simulink model "fm_modulation"  (R2023a)
settings: Solver=VariableStepAuto  StartTime=0.0  StopTime=.1  RelTol=1e-3
settings Model: Creator=USER  LastModifiedBy=USER

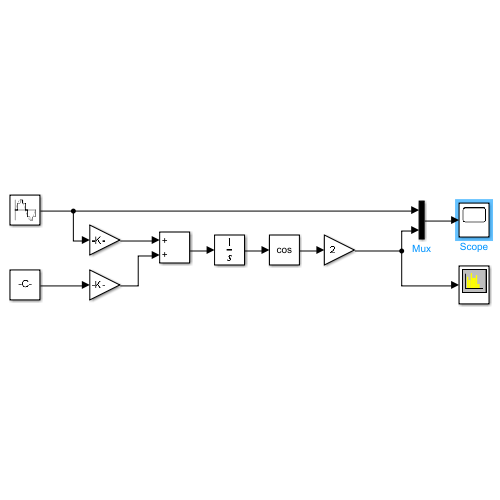
[thumbnail: Simulink's stored preview of the top-level diagram]
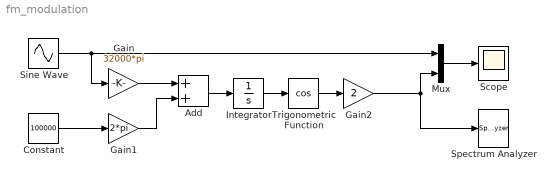
== system fm_modulation ==
  Add : Sum
  Constant : Constant  Value=100000
  Gain : Gain  Gain=32000*pi
  Gain1 : Gain  Gain=2*pi
  Gain2 : Gain  Gain=2
  Integrator : Integrator
  Mux : Mux  Inputs=2
  Scope : Scope
  Sine Wave : Sin  Amplitude=2  Frequency=2*pi*4000  SampleTime=0.000001
  Spectrum Analyzer : SpectrumAnalyzer  WindowPosition=[1.000000,1.000000,1536.000000,841.000000,]  ScopeFrameLocation=window  PlotAsTwoSidedSpectrum=off  Span=5000  CenterFrequency=2500  StartFrequency=0  YLimits=[-75.79047406,34.58708463]  ColorLimits=[-80 20]  SelectedToolstripTab=spectrumAnalyzerToolstrip.spectrumTab
  Trigonometric Function : Trigonometry  Operator=cos
  wires:
  Gain/1 -> Add/1
  Add/1 -> Integrator/1
  Integrator/1 -> Trigonometric Function/1
  Trigonometric Function/1 -> Gain2/1
  Constant/1 -> Gain1/1
  Gain1/1 -> Add/2
  Gain2/1 -> Mux/2, Spectrum Analyzer/1
  Sine Wave/1 -> Gain/1, Mux/1
  Mux/1 -> Scope/1
